simulink model "simu6"  (R2018a)
settings: Solver=VariableStepAuto  StartTime=0.0  StopTime=10.0  RelTol=1e-3
values from neighbouring files (symbols this model uses):
  K_b = 0.1    [DCMotor.m]    (also in exp06matlab.m)
  K_t = 0.1    [DCMotor.m]    (also in exp06matlab.m)
  L = 0.5    [DCMotor.m]    (also in exp06matlab.m)
  R = 1    [DCMotor.m]    (also in exp06matlab.m)
settings Model: Creator=SHRUTI  LastModifiedBy=SHRUTI

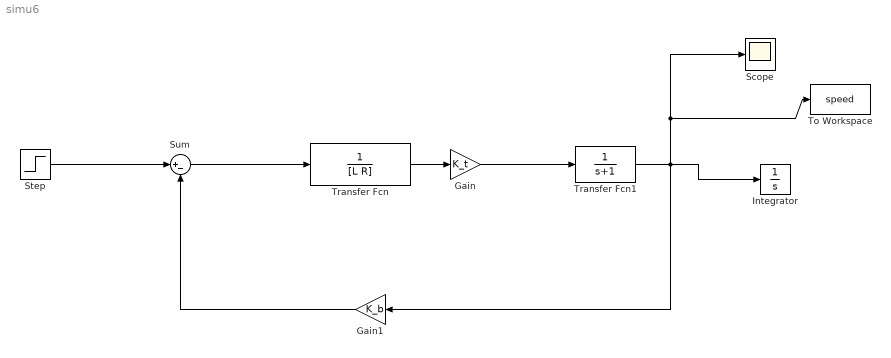
== system simu6 ==
  Gain : Gain  Gain=K_t
  Gain1 : Gain  Gain=K_b
  Integrator : Integrator
  Scope : Scope
  Step : Step  SampleTime=0
  Sum : Sum  Inputs=|+-
  To Workspace : ToWorkspace  VariableName=speed  SampleTime=-1
  Transfer Fcn : TransferFcn  Denominator=[L R]
  Transfer Fcn1 : TransferFcn  Denominator=[1 1]
  wires:
  Step/1 -> Sum/1
  Sum/1 -> Transfer Fcn/1
  Transfer Fcn/1 -> Gain/1
  Gain/1 -> Transfer Fcn1/1
  Gain1/1 -> Sum/2
  Transfer Fcn1/1 -> Gain1/1, To Workspace/1, Scope/1, Integrator/1
